simulink model "controllo_good"  (Simulink 7.9)
settings: Solver=ode45  StartTime=0.0  StopTime=2.0  RelTol=1e-3
values from neighbouring files (symbols this model uses):
  A = [2 3; 4 1]    [ctrl1.m]
  B = [1 0]'    [ctrl1.m]
  C = [1 0]    [ctrl1.m]
  D = 0    [ctrl1.m]
  K = [k1 k2]    [ctrl1.m]
  ueq = 1    [ctrl1.m]
  xeq = -inv(A)*B*ueq    [ctrl1.m]
libraries: simulink x1
settings Model: Creator=patrizio  LastModifiedBy=root
settings DebuggingCC: FcnCallInpInsideContextMsg=Use local settings
settings GRTTargetCC: CombineOutputUpdateFcns=off  GRTInterface=on

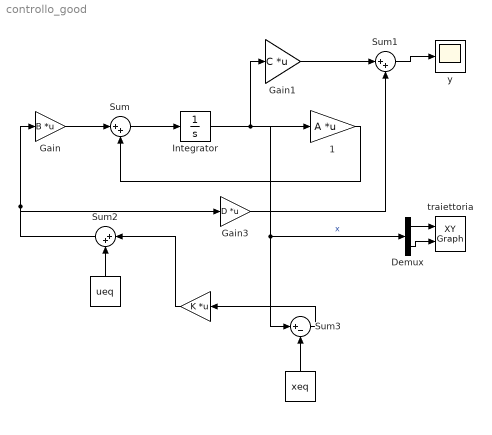
== system controllo_good ==
  " " : Constant  Value=ueq
  "  " : Constant  Value=xeq
  "     " : Gain  Gain=K  Multiplication=Matrix(K*u)
  " 1" : Gain  Gain=A  Multiplication=Matrix(K*u)
  Demux : Demux  Outputs=2
  Gain : Gain  Gain=B  Multiplication=Matrix(K*u)
  Gain1 : Gain  Gain=C  Multiplication=Matrix(K*u)
  Gain3 : Gain  Gain=D  Multiplication=Matrix(K*u)
  Integrator : Integrator
  Sum : Sum  Inputs=|++
  Sum1 : Sum  Inputs=|++
  Sum2 : Sum  Inputs=|++
  Sum3 : Sum  Inputs=|+-
  traiettoria : simulink/Sinks/XY Graph  xmin=-1  xmax=1  ymin=-1  ymax=1  st=-1
  y : Scope
  wires:
  Gain/1 -> Sum/1
  Sum/1 -> Integrator/1
  Integrator/1 -> " 1"/1, Gain1/1, Sum3/1, Demux/1  "x"
  " 1"/1 -> Sum/2
  Gain3/1 -> Sum1/2
  Gain1/1 -> Sum1/1
  " "/1 -> Sum2/2
  "  "/1 -> Sum3/2
  Sum2/1 -> Gain/1, Gain3/1
  Sum1/1 -> y/1
  Demux/1 -> traiettoria/1
  Demux/2 -> traiettoria/2
  Sum3/1 -> "     "/1
  "     "/1 -> Sum2/1
